simulink model "ArmCast_WrapV2_0"  (Simulink 8.2)
settings: Solver=FixedStepDiscrete  StartTime=0.0  StopTime=Inf  RelTol=1e-3
PreLoadFcn:
  | Ts=0.001;
  | Trajectory = load('CastingTrajectory.mat')
undefined symbols (not defined in the file or in its folder): DiscIntNeverNeededParam
libraries: simulink x15, xpclib x7, speedgoatlib_IO102 x4, speedgoatlib_IO301 x4, xpcutilitieslib x3
(part 2 of 2)

== matlab function Controller/State Selection/MATLAB Function ==
  data: state input double; additional_data input double; ud_ar output double; time input double; xd_ar output double; hold_arm output double; ud_sp output double; xd_sp output double; hold_spool output double; armed output double
function [ud_ar, xd_ar, hold_arm, ud_sp, xd_sp, hold_spool, armed] = statemachine(state, additional_data, time)
%#codegen
% This function sends the commands and desired position to the arm and the
% spool.

accu = 10^6;

% Check the additional_data for the correct length
if state == 4
    if size(additional_data, 1) ~= 3
        state = 0;
    end
elseif state == 5
    if size(additional_data, 1) ~= 3
        state = 0;
    end
elseif state == 6
    if size(additional_data, 1) ~= 3
        state = 0;
    end
elseif 0 > sum(state == [2,3])
    if size(additional_data, 1) ~= 1
        state = 0;
    end
end
    

% Initial Values
hold_arm    = false;
hold_spool  = false;
xd_ar       = 0;
ud_ar       = 0;
xd_sp       = 0;
ud_sp       = 0;

% Possible States
switch state
    case 1  %'READY'
        D = coder.load('CastingTrajectory.mat');
        xd_ar   = D.xd_arm(1);
        ud_ar   = D.ud_arm(1);
        xd_sp   = 0;
        ud_sp   = -.5;
        armed   = true;
    case 2  %'ACCEL'
        D = coder.load('CastingTrajectory.mat');
        t       = (time - additional_data(1));   % Mo
        [Val, I]= min(round(accu*abs(D.Time - t))/accu);
        xd_ar   = D.xd_arm(I);
        ud_ar   = D.ud_arm(I);
        xd_sp   = 0;
        ud_sp   = 0;
        armed   = true;
    case 3  %'RELEASE'
        D = coder.load('CastingTrajectory.mat');
        t       = (time - additional_data(1));   % Start Time
        [Val, I]= min(round(accu*abs(D.Time - t))/accu);
        xd_ar   = D.xd_arm(I);
        ud_ar   = D.ud_arm(I);
        xd_sp = 2*pi;
        ud_sp = 6;
        armed = true;
    case 4  %'SPOOL'
        ti  = additional_data(1);   % Initial time
        dxi = additional_data(2);   % Initial x velocity
        dyi = additional_data(3);   % Initial y velocity
        
        t = time - ti;
        x = dxi*t;
        y = dyi*t - 4.905*t^2;
        s = sqrt(x^2 + y^2);
        
        hold_arm = true;
        xp_sp = s*2*pi/(3*.0254) + pi;  % Keep tether at length
        ud_sp = 0;
        
        armed = true;
    case 5  %'WRAP'
        ts  = additional_data(1);   % Start Time
        te  = additional_data(2);   % End Time
        dth = additional_data(3);   % Arm angle rate
        
        if (time < te) && (time < ts)
            D = coder.load('CastingTrajectory.mat');
            t       = (time - additional_data(1));   % Start Time
            [Val, I]= min(round(accu*abs(D.Time - t))/accu);
            pos = D.xd_arm(I) + dth*(time - ts);
        elseif time > te
            D = coder.load('CastingTrajectory.mat');
            t       = (time - additional_data(1));   % Start Time
            [Val, I]= min(round(accu*abs(D.Time - t))/accu);
            pos = D.xd_arm(I) + dth*(te - ts);
        else
            pos = 0;
            hold_arm = true;
        end
            
        xd_ar       = pos;
        ud_ar       = 0;
        hold_spool  = true;
        
        armed = true;
    case 6  %'REARM'
        ts          = additional_data(1);   % Start Time
        arm_init    = additional_data(2);   % Arm starting position
        spool_init  = additional_data(3);   % Spool starting position
        
        t = time - ts;
        
        t_end = spool_init/5;
        
        if t_end > t
            arm_pos = (pi - arm_init)*t/t_end + arm_init;
            spl_pos = spool_init * (1 - t/t_end);
            armed   = true;
        elseif t > t_end
            arm_pos = pi;
            spl_pos = 0;
            armed   = true;
        else
            arm_pos = pi;
            spl_pos = 0;
            armed   = false;
        end
        
        xd_ar   = arm_pos;
        ud_ar   = 0;
        xd_sp   = spl_pos;
        ud_sp   = -1;
    otherwise   %'STOP'
        xd_ar   = 0;
        ud_ar   = 0;
        xd_sp   = 0;
        ud_sp   = 0;
        armed   = false;
end

end

== matlab function FSM/Event Handler/Free Flight Data/Release Velo Calculator ==
  data: enc_data input double; dxdt output double; dydt output double
function [dxdt, dydt]    = RVC(enc_data)
% Release Velocity Calculator, takes the caster state and tranforms it into
% the x and y component velocities of the projectile on release
%#codegen

% enc_data
% 1 Arm pos (rad)
% 2 Arm velo(rad/sec)
% 3 Spool pos (rad)
% 4 Spool velo (rad/sec)
% 5 End Enc pos (rad)
% 6 End Enc velo (rad/sec)
X = enc_data;

h = .438;       % Arm length (m)
l = 11*.0254;   % Rest length (m)
r = (1.5*.0254);  % Spool diameter (m)

th = X(1);
phi= X(5);
R_th    = [cos(th), sin(th); -sin(th), cos(th)];
R_phi   = [cos(phi), sin(phi); -sin(phi), cos(phi)];
dR_th   = [-sin(th), cos(th); -cos(th), -sin(th)];
dR_phi  = [-sin(phi), cos(phi); -cos(phi), -sin(phi)];

% dP = [dxdt,dydt]
dP = X(2)*dR_th*( [0;h] - R_th*[ 0;(l+X(3)*r/pi) ] )...
     - R_th*( X(6)*dR_phi*[ 0;(l+X(3)*r/pi) ] );
 
dxdt = dP(1);
dydt = dP(2);
end

== matlab function FSM/Event Handler/At Goal/MATLAB Function ==
  data: time input double; goal_pos input double; True output boolean; trajectory_data input double
function True = AtGoalCalc(time, goal_pos, trajectory_data)
%#codegen
% Unpackage Trajectory Data
ti  = trajectory_data(1);   % Initial time
dxi = trajectory_data(2);   % Initial x velocity
dyi = trajectory_data(3);   % Initial y velocity

% Position of the projectile relative to the release point
t = time - ti;
x_rel = dxi*t;
y_rel = dyi*t - 4.905*t^2;
a = dyi/dxi;
b = 4.905/dxi^2;

% Vectors for calculating distance to goal
n = [ (a-2*b*x_rel)/sqrt(1+(a-2*b*x_rel)^2);...
       -1/sqrt(1+(a-2*b*x_rel)^2) ];
c = [x_rel; y_rel];
d = [goal_pos(1); goal_pos(2)];

p = (c-d) - ( dot((c-d),n) )*n;

True = false;
% Event if negative y velocity and line close to the goal
True = and( ((a-2*b*x_rel) < 0) , ( sqrt(p(1)^2 + p(2)^2) < 0.15) );
end

== matlab function FSM/Event Handler/Free Flight Data/Goal Position Calculator ==
  data: enc_data input double; x output double; y output double
function [x, y] = GPC(enc_data)
% Goal Position Calculator, takes the caster state and calculates the
% position of the goal relative to the release point.  The x and y 
% component is the position of said goal.
%#codegen

% enc_data
% 1 Arm pos (rad)
% 2 Arm velo(rad/sec)
% 3 Spool pos (rad)
% 4 Spool velo (rad/sec)
% 5 End Enc pos (rad)
% 6 End Enc velo (rad/sec)

% Constants
% Goal position relative to the pivot of the arm
Gx  = 2.415;
Gy  = 0.21;
h   = .438;       % Arm length (m)
l   = 11*.0254;   % Rest length (m) of tether
d   = (1.5*.0254);  % Spool diameter (m)

th = enc_data(1);
phi= enc_data(5);
R_th    = [cos(th), sin(th); -sin(th), cos(th)];
R_phi   = [cos(phi), sin(phi); -sin(phi), cos(phi)];

% P = [x, y]'
P = R_th*( [0;h] - R_phi*[0;l] );
 
x = P(1);
y = P(2);

end

== matlab function FSM/Event Handler/State Selection ==
  data: Events input double; state output double; previous input double
function state = StateSelector(Events, previous)
% State Selector, input is events and previous states.  Processes this data
% to determine which state the system should presently be in.
%#codegen

% Events
% 1 Fire == true
% 2 Release == true
% 3 Free Flight Check == true
% 4 At Goal == true
% 5 Wrap Done == true
% 6 Re-arm == true
% 7 Reset Done == true
% 8 Safety == true

% Previous State

% Initialize, if it doesn't get the signal, it doesn't change.
state = previous;

% State selector
switch previous
    case 1  %'READY'
        if Events(1) % 'fire'
            state = 2;
        end
    case 2  %'ACCEL'
        if Events(2) % 'release'
            state = 3;
        end
    case 3  %'RELEASE'
        if Events(3) % 'free flight check'
            state = 4;
        end
    case 4  %'SPOOL'
        if Events(4) % 'at goal'
            state = 5;
        end
    case 5  %'WRAP'
        if Events(5) % 'wrap done'
            state = 0;
        end
    case 6  %'REARM'
        if Events(7) % 'reset done'
            state = 1;
        end
    otherwise   %'STOP' 0th state
        if Events(6) % 're-arm'
            state = 6;
        else
            state = 0;
        end
end

% Send Robot to Stopped State if we ever recieve the safety signal
if Events(8) % 'safety'
    state = 0;
end

end
